simulink model "canPack_BCU_09"  (R2020a)
settings: Solver=VariableStepAuto  StartTime=0.0  StopTime=10.0  RelTol=1e-3
libraries: MyLibrary x1
settings Model: Creator=Administrator  LastModifiedBy=Administrator

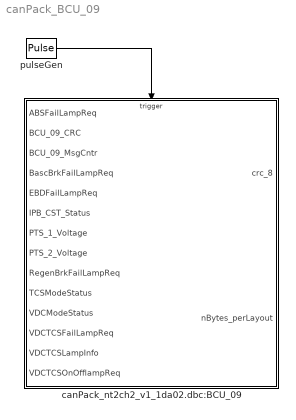
== system canPack_BCU_09 ==
  canPack_nt2ch2_v1_1da02.dbc:BCU_09 : Subsystem
  pulseGen : DiscretePulseGenerator  PulseType=Time based  Period=0.1  PulseWidth=50
  wires:
  pulseGen/1 -> canPack_nt2ch2_v1_1da02.dbc:BCU_09/Trigger

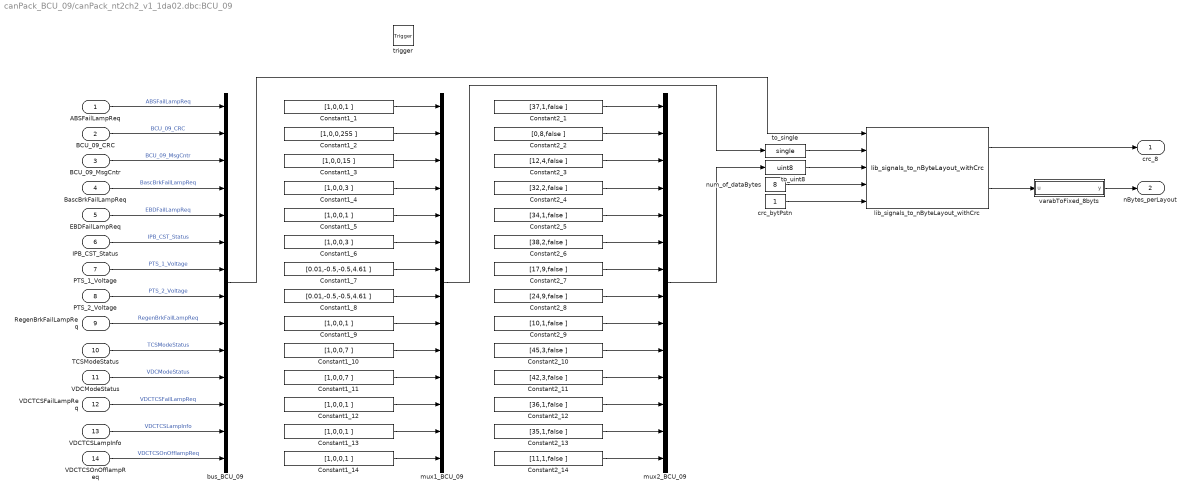
== system canPack_BCU_09/canPack_nt2ch2_v1_1da02.dbc:BCU_09 ==
  ABSFailLampReq : Inport
  BCU_09_CRC : Inport  Port=2
  BCU_09_MsgCntr : Inport  Port=3
  BascBrkFailLampReq : Inport  Port=4
  EBDFailLampReq : Inport  Port=5
  IPB_CST_Status : Inport  Port=6
  PTS_1_Voltage : Inport  Port=7
  PTS_2_Voltage : Inport  Port=8
  RegenBrkFailLampReq : Inport  Port=9
  TCSModeStatus : Inport  Port=10
  VDCModeStatus : Inport  Port=11
  VDCTCSFailLampReq : Inport  Port=12
  VDCTCSLampInfo : Inport  Port=13
  VDCTCSOnOfflampReq : Inport  Port=14
  trigger : TriggerPort  TriggerType=either  VariantControl=Variant  PortDimensions=1
  Constant1_{1,5,9,12..14} (6 alike) : Constant  Value=[1,0,0,1 ]  SampleTime=-1
  Constant1_10 : Constant  Value=[1,0,0,7 ]  SampleTime=-1
  Constant1_11 : Constant  Value=[1,0,0,7 ]  SampleTime=-1
  Constant1_2 : Constant  Value=[1,0,0,255 ]  SampleTime=-1
  Constant1_3 : Constant  Value=[1,0,0,15 ]  SampleTime=-1
  Constant1_4 : Constant  Value=[1,0,0,3 ]  SampleTime=-1
  Constant1_6 : Constant  Value=[1,0,0,3 ]  SampleTime=-1
  Constant1_7 : Constant  Value=[0.01,-0.5,-0.5,4.61 ]  SampleTime=-1
  Constant1_8 : Constant  Value=[0.01,-0.5,-0.5,4.61 ]  SampleTime=-1
  Constant2_1 : Constant  Value=[37,1,false ]  SampleTime=-1
  Constant2_10 : Constant  Value=[45,3,false ]  SampleTime=-1
  Constant2_11 : Constant  Value=[42,3,false ]  SampleTime=-1
  Constant2_12 : Constant  Value=[36,1,false ]  SampleTime=-1
  Constant2_13 : Constant  Value=[35,1,false ]  SampleTime=-1
  Constant2_14 : Constant  Value=[11,1,false ]  SampleTime=-1
  Constant2_2 : Constant  Value=[0,8,false ]  SampleTime=-1
  Constant2_3 : Constant  Value=[12,4,false ]  SampleTime=-1
  Constant2_4 : Constant  Value=[32,2,false ]  SampleTime=-1
  Constant2_5 : Constant  Value=[34,1,false ]  SampleTime=-1
  Constant2_6 : Constant  Value=[38,2,false ]  SampleTime=-1
  Constant2_7 : Constant  Value=[17,9,false ]  SampleTime=-1
  Constant2_8 : Constant  Value=[24,9,false ]  SampleTime=-1
  Constant2_9 : Constant  Value=[10,1,false ]  SampleTime=-1
  bus_BCU_09 : BusCreator  Inputs=14
  crc_bytPstn : Constant  OutDataTypeStr=uint8  SampleTime=-1
  lib_signals_to_nByteLayout_withCrc : MyLibrary/lib_signals_to_nByteLayout_withCrc  SystemSampleTime=-1  Latency=0  AutoFrameSizeCalculation=off
  mux1_BCU_09 : Mux  Inputs=14
  mux2_BCU_09 : Mux  Inputs=14
  num_of_dataBytes : Constant  Value=8  OutDataTypeStr=uint8  SampleTime=-1
  to_single : DataTypeConversion  OutDataTypeStr=single
  to_uint8 : DataTypeConversion  OutDataTypeStr=uint8
  varabToFixed_8byts : MATLAB Function  TreatAsAtomicUnit=on
  crc_8 : Outport
  nBytes_perLayout : Outport  Port=2
  wires:
  ABSFailLampReq/1 -> bus_BCU_09/1  "ABSFailLampReq"
  BCU_09_CRC/1 -> bus_BCU_09/2  "BCU_09_CRC"
  BCU_09_MsgCntr/1 -> bus_BCU_09/3  "BCU_09_MsgCntr"
  BascBrkFailLampReq/1 -> bus_BCU_09/4  "BascBrkFailLampReq"
  EBDFailLampReq/1 -> bus_BCU_09/5  "EBDFailLampReq"
  IPB_CST_Status/1 -> bus_BCU_09/6  "IPB_CST_Status"
  PTS_1_Voltage/1 -> bus_BCU_09/7  "PTS_1_Voltage"
  PTS_2_Voltage/1 -> bus_BCU_09/8  "PTS_2_Voltage"
  RegenBrkFailLampReq/1 -> bus_BCU_09/9  "RegenBrkFailLampReq"
  TCSModeStatus/1 -> bus_BCU_09/10  "TCSModeStatus"
  VDCModeStatus/1 -> bus_BCU_09/11  "VDCModeStatus"
  VDCTCSFailLampReq/1 -> bus_BCU_09/12  "VDCTCSFailLampReq"
  VDCTCSLampInfo/1 -> bus_BCU_09/13  "VDCTCSLampInfo"
  VDCTCSOnOfflampReq/1 -> bus_BCU_09/14  "VDCTCSOnOfflampReq"
  Constant1_1/1 -> mux1_BCU_09/1
  Constant2_1/1 -> mux2_BCU_09/1
  Constant1_2/1 -> mux1_BCU_09/2
  Constant2_2/1 -> mux2_BCU_09/2
  Constant1_3/1 -> mux1_BCU_09/3
  Constant2_3/1 -> mux2_BCU_09/3
  Constant1_4/1 -> mux1_BCU_09/4
  Constant2_4/1 -> mux2_BCU_09/4
  Constant1_5/1 -> mux1_BCU_09/5
  Constant2_5/1 -> mux2_BCU_09/5
  Constant1_6/1 -> mux1_BCU_09/6
  Constant2_6/1 -> mux2_BCU_09/6
  Constant1_7/1 -> mux1_BCU_09/7
  Constant2_7/1 -> mux2_BCU_09/7
  Constant1_8/1 -> mux1_BCU_09/8
  Constant2_8/1 -> mux2_BCU_09/8
  Constant1_9/1 -> mux1_BCU_09/9
  Constant2_9/1 -> mux2_BCU_09/9
  Constant1_10/1 -> mux1_BCU_09/10
  Constant2_10/1 -> mux2_BCU_09/10
  Constant1_11/1 -> mux1_BCU_09/11
  Constant2_11/1 -> mux2_BCU_09/11
  Constant1_12/1 -> mux1_BCU_09/12
  Constant2_12/1 -> mux2_BCU_09/12
  Constant1_13/1 -> mux1_BCU_09/13
  Constant2_13/1 -> mux2_BCU_09/13
  Constant1_14/1 -> mux1_BCU_09/14
  Constant2_14/1 -> mux2_BCU_09/14
  bus_BCU_09/1 -> lib_signals_to_nByteLayout_withCrc/1
  mux1_BCU_09/1 -> to_single/1
  to_single/1 -> lib_signals_to_nByteLayout_withCrc/2
  mux2_BCU_09/1 -> to_uint8/1
  to_uint8/1 -> lib_signals_to_nByteLayout_withCrc/3
  lib_signals_to_nByteLayout_withCrc/1 -> crc_8/1
  num_of_dataBytes/1 -> lib_signals_to_nByteLayout_withCrc/4
  lib_signals_to_nByteLayout_withCrc/2 -> varabToFixed_8byts/1(u)
  varabToFixed_8byts/1(y) -> nBytes_perLayout/1
  crc_bytPstn/1 -> lib_signals_to_nByteLayout_withCrc/5

== matlab function canPack_BCU_09/canPack_nt2ch2_v1_1da02.dbc:BCU_09/varabToFixed_8byts ==
  data: u input uint8 size=8; y output uint8
function y = fcn(u)

fixed_size = 8;
y = uint8(zeros(fixed_size,1));

for i=1:fixed_size
    y(i) = u(i);
end
